simulink model "sevietta_devel_2017h"  (R2013a)
(part 6 of 31)

      | % if (strcmp(mode, 'one value') || strcmp(mode, 'fields of equal size')) && (length(current_widths) > 1),
      | %     error('Only one width may be specified for this mode.');
      | % elseif strcmp(mode, 'fields of arbitrary size')
      | %     current_names = textscan(strtrim(strrep(strrep(get_param(blk, 'names'), ']', ''), '[', '')), '%s');
      | %     current_names = current_names{1};
      | %     numios = length(current_names);
      | %     if length(current_widths) ~= numios,
      | %         error('%d field names specified, but %d widths?', numios, length(current_widths));
      | %     end
      | % end
      | % total_width = 0;
      | % for ctr = 1 : length(current_widths),
      | %     total_width = total_width + current_widths(ctr);
      | % end
      | % if total_width > 32,
      | %     error('Total width must be 32 or less, set to %d.', total_width);
      | % end
      mask Callback arith_types:
      | [numios, ~, ~, ~, current_types] = swreg_maskcheck(gcb);
      | % blk = gcb;
      | % mode = get_param(blk, 'mode');
      | % current_types = eval(get_param(blk, 'arith_types'));
      | % numios = length(current_types);
      | % if (strcmp(mode, 'one value') || strcmp(mode, 'fields of equal size')) && (length(current_types) > 1),
      | %     error('Only one type may be specified for this mode.');
      | % elseif strcmp(mode, 'fields of arbitrary size')
      | %     current_names = textscan(strtrim(strrep(strrep(get_param(blk, 'names'), ']', ''), '[', '')), '%s');
      | %     current_names = current_names{1};
      | %     numios = length(current_names);
      | %     if length(current_types) ~= numios,
      | %         error('%d field names specified, but %d types?', numios, length(current_types));
      | %     end
      | % end
      | problem = 0;
      | for ctr = 1 : numios,
      |     t = current_types(ctr);
      |     if (t < 0) || (t > 2),
      |         problem = t;
      |         ctr = numios + 1;
      |     end
      | end
      | if problem ~= 0,
      |     error('Type cannot be %i, must be 0, 1 or 2.', problem);
      | end
      mask Callback bin_pts:
      | swreg_maskcheck(gcb);
      | % blk = gcb;
      | % mode = get_param(blk, 'mode');
      | % current_bins = eval(get_param(blk, 'bin_pts'));
      | % if (strcmp(mode, 'one value') || strcmp(mode, 'fields of equal size')) && (length(current_bins) > 1),
      | %     error('Only one binary pt may be specified for this mode.');
      | % elseif strcmp(mode, 'fields of arbitrary size')
      | %     current_names = textscan(strtrim(strrep(strrep(get_param(blk, 'names'), ']', ''), '[', '')), '%s');
      | %     current_names = current_names{1};
      | %     numios = length(current_names);
      | %     if length(current_bins) ~= numios,
      | %         error('%d field names specified, but %d binary pts?', numios, length(current_bins));
      | %     end
      | % end
  packetizer : Subsystem
  packetizer1 : Subsystem
  packetizer2 : Subsystem
  packetizer3 : Subsystem
  pipeline1 : Subsystem  AncestorBlock=casper_library_delays/pipeline  mask(pipeline){latency=1}
      mask help:
      | An explicitly laid-out delay line to avoid mapping to SRL16s
      | for use in pipelining to help achieve timing closure.
      mask init:
      | pipeline_init(gcb,'latency',latency);
      settings: AttributesFormatString=Latency = %<latency>
      mask Display:
      | port_label('input', 1, 'd');
      | port_label('output', 1, 'q');
      | disp(['Z^-', num2str(latency)]);
  pipeline10 : Subsystem  AncestorBlock=casper_library_delays/pipeline  mask(pipeline){latency=1}
      mask help:
      | An explicitly laid-out delay line to avoid mapping to SRL16s
      | for use in pipelining to help achieve timing closure.
      mask init:
      | pipeline_init(gcb,'latency',latency);
      settings: AttributesFormatString=Latency = %<latency>
      mask Display:
      | port_label('input', 1, 'd');
      | port_label('output', 1, 'q');
      | disp(['Z^-', num2str(latency)]);
  pipeline11 : Subsystem  AncestorBlock=casper_library_delays/pipeline  mask(pipeline){latency=1}
      mask help:
      | An explicitly laid-out delay line to avoid mapping to SRL16s
      | for use in pipelining to help achieve timing closure.
      mask init:
      | pipeline_init(gcb,'latency',latency);
      settings: AttributesFormatString=Latency = %<latency>
      mask Display:
      | port_label('input', 1, 'd');
      | port_label('output', 1, 'q');
      | disp(['Z^-', num2str(latency)]);
  pipeline12 : Subsystem  AncestorBlock=casper_library_delays/pipeline  mask(pipeline){latency=1}
      mask help:
      | An explicitly laid-out delay line to avoid mapping to SRL16s
      | for use in pipelining to help achieve timing closure.
      mask init:
      | pipeline_init(gcb,'latency',latency);
      settings: AttributesFormatString=Latency = %<latency>
      mask Display:
      | port_label('input', 1, 'd');
      | port_label('output', 1, 'q');
      | disp(['Z^-', num2str(latency)]);
  pipeline13 : Subsystem  AncestorBlock=casper_library_delays/pipeline  mask(pipeline){latency=1}
      mask help:
      | An explicitly laid-out delay line to avoid mapping to SRL16s
      | for use in pipelining to help achieve timing closure.
      mask init:
      | pipeline_init(gcb,'latency',latency);
      settings: AttributesFormatString=Latency = %<latency>
      mask Display:
      | port_label('input', 1, 'd');
      | port_label('output', 1, 'q');
      | disp(['Z^-', num2str(latency)]);
  pipeline14 : Subsystem  AncestorBlock=casper_library_delays/pipeline  mask(pipeline){latency=1}
      mask help:
      | An explicitly laid-out delay line to avoid mapping to SRL16s
      | for use in pipelining to help achieve timing closure.
      mask init:
      | pipeline_init(gcb,'latency',latency);
      settings: AttributesFormatString=Latency = %<latency>
      mask Display:
      | port_label('input', 1, 'd');
      | port_label('output', 1, 'q');
      | disp(['Z^-', num2str(latency)]);
  pipeline15 : Subsystem  AncestorBlock=casper_library_delays/pipeline  mask(pipeline){latency=1}
      mask help:
      | An explicitly laid-out delay line to avoid mapping to SRL16s
      | for use in pipelining to help achieve timing closure.
      mask init:
      | pipeline_init(gcb,'latency',latency);
      settings: AttributesFormatString=Latency = %<latency>
      mask Display:
      | port_label('input', 1, 'd');
      | port_label('output', 1, 'q');
      | disp(['Z^-', num2str(latency)]);
  pipeline16 : Subsystem  AncestorBlock=casper_library_delays/pipeline  mask(pipeline){latency=1}
      mask help:
      | An explicitly laid-out delay line to avoid mapping to SRL16s
      | for use in pipelining to help achieve timing closure.
      mask init:
      | pipeline_init(gcb,'latency',latency);
      settings: AttributesFormatString=Latency = %<latency>
      mask Display:
      | port_label('input', 1, 'd');
      | port_label('output', 1, 'q');
      | disp(['Z^-', num2str(latency)]);
  pipeline17 : Subsystem  AncestorBlock=casper_library_delays/pipeline  mask(pipeline){latency=1}
      mask help:
      | An explicitly laid-out delay line to avoid mapping to SRL16s
      | for use in pipelining to help achieve timing closure.
      mask init:
      | pipeline_init(gcb,'latency',latency);
      settings: AttributesFormatString=Latency = %<latency>
      mask Display:
      | port_label('input', 1, 'd');
      | port_label('output', 1, 'q');
      | disp(['Z^-', num2str(latency)]);
  pipeline18 : Subsystem  AncestorBlock=casper_library_delays/pipeline  mask(pipeline){latency=1}
      mask help:
      | An explicitly laid-out delay line to avoid mapping to SRL16s
      | for use in pipelining to help achieve timing closure.
      mask init:
      | pipeline_init(gcb,'latency',latency);
      settings: AttributesFormatString=Latency = %<latency>
      mask Display:
      | port_label('input', 1, 'd');
      | port_label('output', 1, 'q');
      | disp(['Z^-', num2str(latency)]);
  pipeline19 : Subsystem  AncestorBlock=casper_library_delays/pipeline  mask(pipeline){latency=1}
      mask help:
      | An explicitly laid-out delay line to avoid mapping to SRL16s
      | for use in pipelining to help achieve timing closure.
      mask init:
      | pipeline_init(gcb,'latency',latency);
      settings: AttributesFormatString=Latency = %<latency>
      mask Display:
      | port_label('input', 1, 'd');
      | port_label('output', 1, 'q');
      | disp(['Z^-', num2str(latency)]);
  pipeline2 : Subsystem  AncestorBlock=casper_library_delays/pipeline  mask(pipeline){latency=1}
      mask help:
      | An explicitly laid-out delay line to avoid mapping to SRL16s
      | for use in pipelining to help achieve timing closure.
      mask init:
      | pipeline_init(gcb,'latency',latency);
      settings: AttributesFormatString=Latency = %<latency>
      mask Display:
      | port_label('input', 1, 'd');
      | port_label('output', 1, 'q');
      | disp(['Z^-', num2str(latency)]);
  pipeline20 : Subsystem  AncestorBlock=casper_library_delays/pipeline  mask(pipeline){latency=1}
      mask help:
      | An explicitly laid-out delay line to avoid mapping to SRL16s
      | for use in pipelining to help achieve timing closure.
      mask init:
      | pipeline_init(gcb,'latency',latency);
      settings: AttributesFormatString=Latency = %<latency>
      mask Display:
      | port_label('input', 1, 'd');
      | port_label('output', 1, 'q');
      | disp(['Z^-', num2str(latency)]);
  pipeline21 : Subsystem  AncestorBlock=casper_library_delays/pipeline  mask(pipeline){latency=1}
      mask help:
      | An explicitly laid-out delay line to avoid mapping to SRL16s
      | for use in pipelining to help achieve timing closure.
      mask init:
      | pipeline_init(gcb,'latency',latency);
      settings: AttributesFormatString=Latency = %<latency>
      mask Display:
      | port_label('input', 1, 'd');
      | port_label('output', 1, 'q');
      | disp(['Z^-', num2str(latency)]);
  pipeline22 : Subsystem  AncestorBlock=casper_library_delays/pipeline  mask(pipeline){latency=1}
      mask help:
      | An explicitly laid-out delay line to avoid mapping to SRL16s
      | for use in pipelining to help achieve timing closure.
      mask init:
      | pipeline_init(gcb,'latency',latency);
      settings: AttributesFormatString=Latency = %<latency>
      mask Display:
      | port_label('input', 1, 'd');
      | port_label('output', 1, 'q');
      | disp(['Z^-', num2str(latency)]);
  pipeline23 : Subsystem  AncestorBlock=casper_library_delays/pipeline  mask(pipeline){latency=1}
      mask help:
      | An explicitly laid-out delay line to avoid mapping to SRL16s
      | for use in pipelining to help achieve timing closure.
      mask init:
      | pipeline_init(gcb,'latency',latency);
      settings: AttributesFormatString=Latency = %<latency>
      mask Display:
      | port_label('input', 1, 'd');
      | port_label('output', 1, 'q');
      | disp(['Z^-', num2str(latency)]);
  pipeline24 : Subsystem  AncestorBlock=casper_library_delays/pipeline  mask(pipeline){latency=1}
      mask help:
      | An explicitly laid-out delay line to avoid mapping to SRL16s
      | for use in pipelining to help achieve timing closure.
      mask init:
      | pipeline_init(gcb,'latency',latency);
      settings: AttributesFormatString=Latency = %<latency>
      mask Display:
      | port_label('input', 1, 'd');
      | port_label('output', 1, 'q');
      | disp(['Z^-', num2str(latency)]);
  pipeline25 : Subsystem  AncestorBlock=casper_library_delays/pipeline  mask(pipeline){latency=1}
      mask help:
      | An explicitly laid-out delay line to avoid mapping to SRL16s
      | for use in pipelining to help achieve timing closure.
      mask init:
      | pipeline_init(gcb,'latency',latency);
      settings: AttributesFormatString=Latency = %<latency>
      mask Display:
      | port_label('input', 1, 'd');
      | port_label('output', 1, 'q');
      | disp(['Z^-', num2str(latency)]);
  pipeline26 : Subsystem  AncestorBlock=casper_library_delays/pipeline  mask(pipeline){latency=1}
      mask help:
      | An explicitly laid-out delay line to avoid mapping to SRL16s
      | for use in pipelining to help achieve timing closure.
      mask init:
      | pipeline_init(gcb,'latency',latency);
      settings: AttributesFormatString=Latency = %<latency>
      mask Display:
      | port_label('input', 1, 'd');
      | port_label('output', 1, 'q');
      | disp(['Z^-', num2str(latency)]);
  pipeline27 : Subsystem  AncestorBlock=casper_library_delays/pipeline  mask(pipeline){latency=1}
      mask help:
      | An explicitly laid-out delay line to avoid mapping to SRL16s
      | for use in pipelining to help achieve timing closure.
      mask init:
      | pipeline_init(gcb,'latency',latency);
      settings: AttributesFormatString=Latency = %<latency>
      mask Display:
      | port_label('input', 1, 'd');
      | port_label('output', 1, 'q');
      | disp(['Z^-', num2str(latency)]);
  pipeline28 : Subsystem  AncestorBlock=casper_library_delays/pipeline  mask(pipeline){latency=1}
      mask help:
      | An explicitly laid-out delay line to avoid mapping to SRL16s
      | for use in pipelining to help achieve timing closure.
      mask init:
      | pipeline_init(gcb,'latency',latency);
      settings: AttributesFormatString=Latency = %<latency>
      mask Display:
      | port_label('input', 1, 'd');
      | port_label('output', 1, 'q');
      | disp(['Z^-', num2str(latency)]);
  pipeline29 : Subsystem  AncestorBlock=casper_library_delays/pipeline  mask(pipeline){latency=1}
      mask help:
      | An explicitly laid-out delay line to avoid mapping to SRL16s
      | for use in pipelining to help achieve timing closure.
      mask init:
      | pipeline_init(gcb,'latency',latency);
      settings: AttributesFormatString=Latency = %<latency>
      mask Display:
      | port_label('input', 1, 'd');
      | port_label('output', 1, 'q');
      | disp(['Z^-', num2str(latency)]);
  pipeline3 : Subsystem  AncestorBlock=casper_library_delays/pipeline  mask(pipeline){latency=1}
      mask help:
      | An explicitly laid-out delay line to avoid mapping to SRL16s
      | for use in pipelining to help achieve timing closure.
      mask init:
      | pipeline_init(gcb,'latency',latency);
      settings: AttributesFormatString=Latency = %<latency>
      mask Display:
      | port_label('input', 1, 'd');
      | port_label('output', 1, 'q');
      | disp(['Z^-', num2str(latency)]);
  pipeline30 : Subsystem  AncestorBlock=casper_library_delays/pipeline  mask(pipeline){latency=1}
      mask help:
      | An explicitly laid-out delay line to avoid mapping to SRL16s
      | for use in pipelining to help achieve timing closure.
      mask init:
      | pipeline_init(gcb,'latency',latency);
      settings: AttributesFormatString=Latency = %<latency>
      mask Display:
      | port_label('input', 1, 'd');
      | port_label('output', 1, 'q');
      | disp(['Z^-', num2str(latency)]);
  pipeline31 : Subsystem  AncestorBlock=casper_library_delays/pipeline  mask(pipeline){latency=1}
      mask help:
      | An explicitly laid-out delay line to avoid mapping to SRL16s
      | for use in pipelining to help achieve timing closure.
      mask init:
      | pipeline_init(gcb,'latency',latency);
      settings: AttributesFormatString=Latency = %<latency>
      mask Display:
      | port_label('input', 1, 'd');
      | port_label('output', 1, 'q');
      | disp(['Z^-', num2str(latency)]);
  pipeline32 : Subsystem  AncestorBlock=casper_library_delays/pipeline  mask(pipeline){latency=1}
      mask help:
      | An explicitly laid-out delay line to avoid mapping to SRL16s
      | for use in pipelining to help achieve timing closure.
      mask init:
      | pipeline_init(gcb,'latency',latency);
      settings: AttributesFormatString=Latency = %<latency>
      mask Display:
      | port_label('input', 1, 'd');
      | port_label('output', 1, 'q');
      | disp(['Z^-', num2str(latency)]);
  pipeline33 : Subsystem  AncestorBlock=casper_library_delays/pipeline  mask(pipeline){latency=1}
      mask help:
      | An explicitly laid-out delay line to avoid mapping to SRL16s
      | for use in pipelining to help achieve timing closure.
      mask init:
      | pipeline_init(gcb,'latency',latency);
      settings: AttributesFormatString=Latency = %<latency>
      mask Display:
      | port_label('input', 1, 'd');
      | port_label('output', 1, 'q');
      | disp(['Z^-', num2str(latency)]);
  pipeline34 : Subsystem  AncestorBlock=casper_library_delays/pipeline  mask(pipeline){latency=1}
      mask help:
      | An explicitly laid-out delay line to avoid mapping to SRL16s
      | for use in pipelining to help achieve timing closure.
      mask init:
      | pipeline_init(gcb,'latency',latency);
      settings: AttributesFormatString=Latency = %<latency>
      mask Display:
      | port_label('input', 1, 'd');
      | port_label('output', 1, 'q');
      | disp(['Z^-', num2str(latency)]);
  pipeline35 : Subsystem  AncestorBlock=casper_library_delays/pipeline  mask(pipeline){latency=1}
      mask help:
      | An explicitly laid-out delay line to avoid mapping to SRL16s
      | for use in pipelining to help achieve timing closure.
      mask init:
      | pipeline_init(gcb,'latency',latency);
      settings: AttributesFormatString=Latency = %<latency>
      mask Display:
      | port_label('input', 1, 'd');
      | port_label('output', 1, 'q');
      | disp(['Z^-', num2str(latency)]);
  pipeline36 : Subsystem  AncestorBlock=casper_library_delays/pipeline  mask(pipeline){latency=1}
      mask help:
      | An explicitly laid-out delay line to avoid mapping to SRL16s
      | for use in pipelining to help achieve timing closure.
      mask init:
      | pipeline_init(gcb,'latency',latency);
      settings: AttributesFormatString=Latency = %<latency>
      mask Display:
      | port_label('input', 1, 'd');
      | port_label('output', 1, 'q');
      | disp(['Z^-', num2str(latency)]);
  pipeline37 : Subsystem  AncestorBlock=casper_library_delays/pipeline  mask(pipeline){latency=1}
      mask help:
      | An explicitly laid-out delay line to avoid mapping to SRL16s
      | for use in pipelining to help achieve timing closure.
      mask init:
      | pipeline_init(gcb,'latency',latency);
      settings: AttributesFormatString=Latency = %<latency>
      mask Display:
      | port_label('input', 1, 'd');
      | port_label('output', 1, 'q');
      | disp(['Z^-', num2str(latency)]);
  pipeline38 : Subsystem  AncestorBlock=casper_library_delays/pipeline  mask(pipeline){latency=1}
      mask help:
      | An explicitly laid-out delay line to avoid mapping to SRL16s
      | for use in pipelining to help achieve timing closure.
      mask init:
      | pipeline_init(gcb,'latency',latency);
      settings: AttributesFormatString=Latency = %<latency>
      mask Display:
      | port_label('input', 1, 'd');
      | port_label('output', 1, 'q');
      | disp(['Z^-', num2str(latency)]);
  pipeline39 : Subsystem  AncestorBlock=casper_library_delays/pipeline  mask(pipeline){latency=1}
      mask help:
      | An explicitly laid-out delay line to avoid mapping to SRL16s
      | for use in pipelining to help achieve timing closure.
      mask init:
      | pipeline_init(gcb,'latency',latency);
      settings: AttributesFormatString=Latency = %<latency>
      mask Display:
      | port_label('input', 1, 'd');
      | port_label('output', 1, 'q');
      | disp(['Z^-', num2str(latency)]);
  pipeline4 : Subsystem  AncestorBlock=casper_library_delays/pipeline  mask(pipeline){latency=1}
      mask help:
      | An explicitly laid-out delay line to avoid mapping to SRL16s
      | for use in pipelining to help achieve timing closure.
      mask init:
      | pipeline_init(gcb,'latency',latency);
      settings: AttributesFormatString=Latency = %<latency>
      mask Display:
      | port_label('input', 1, 'd');
      | port_label('output', 1, 'q');
      | disp(['Z^-', num2str(latency)]);
  pipeline40 : Subsystem  AncestorBlock=casper_library_delays/pipeline  mask(pipeline){latency=1}
      mask help:
      | An explicitly laid-out delay line to avoid mapping to SRL16s
      | for use in pipelining to help achieve timing closure.
      mask init:
      | pipeline_init(gcb,'latency',latency);
      settings: AttributesFormatString=Latency = %<latency>
      mask Display:
      | port_label('input', 1, 'd');
      | port_label('output', 1, 'q');
      | disp(['Z^-', num2str(latency)]);
  pipeline41 : Subsystem  AncestorBlock=casper_library_delays/pipeline  mask(pipeline){latency=1}
      mask help:
      | An explicitly laid-out delay line to avoid mapping to SRL16s
      | for use in pipelining to help achieve timing closure.
      mask init:
      | pipeline_init(gcb,'latency',latency);
      settings: AttributesFormatString=Latency = %<latency>
      mask Display:
      | port_label('input', 1, 'd');
      | port_label('output', 1, 'q');
      | disp(['Z^-', num2str(latency)]);
  pipeline42 : Subsystem  AncestorBlock=casper_library_delays/pipeline  mask(pipeline){latency=1}
      mask help:
      | An explicitly laid-out delay line to avoid mapping to SRL16s
      | for use in pipelining to help achieve timing closure.
      mask init:
      | pipeline_init(gcb,'latency',latency);
      settings: AttributesFormatString=Latency = %<latency>
      mask Display:
      | port_label('input', 1, 'd');
      | port_label('output', 1, 'q');
      | disp(['Z^-', num2str(latency)]);
  pipeline43 : Subsystem  AncestorBlock=casper_library_delays/pipeline  mask(pipeline){latency=1}
      mask help:
      | An explicitly laid-out delay line to avoid mapping to SRL16s
      | for use in pipelining to help achieve timing closure.
      mask init:
      | pipeline_init(gcb,'latency',latency);
      settings: AttributesFormatString=Latency = %<latency>
      mask Display:
      | port_label('input', 1, 'd');
      | port_label('output', 1, 'q');
      | disp(['Z^-', num2str(latency)]);
  pipeline44 : Subsystem  AncestorBlock=casper_library_delays/pipeline  mask(pipeline){latency=1}
      mask help:
      | An explicitly laid-out delay line to avoid mapping to SRL16s
      | for use in pipelining to help achieve timing closure.
      mask init:
      | pipeline_init(gcb,'latency',latency);
      settings: AttributesFormatString=Latency = %<latency>
      mask Display:
      | port_label('input', 1, 'd');
      | port_label('output', 1, 'q');
      | disp(['Z^-', num2str(latency)]);
  pipeline45 : Subsystem  AncestorBlock=casper_library_delays/pipeline  mask(pipeline){latency=1}
      mask help:
      | An explicitly laid-out delay line to avoid mapping to SRL16s
      | for use in pipelining to help achieve timing closure.
      mask init:
      | pipeline_init(gcb,'latency',latency);
      settings: AttributesFormatString=Latency = %<latency>
      mask Display:
      | port_label('input', 1, 'd');
      | port_label('output', 1, 'q');
      | disp(['Z^-', num2str(latency)]);
  pipeline46 : Subsystem  AncestorBlock=casper_library_delays/pipeline  mask(pipeline){latency=1}
      mask help:
      | An explicitly laid-out delay line to avoid mapping to SRL16s
      | for use in pipelining to help achieve timing closure.
      mask init:
      | pipeline_init(gcb,'latency',latency);
      settings: AttributesFormatString=Latency = %<latency>
      mask Display:
      | port_label('input', 1, 'd');
      | port_label('output', 1, 'q');
      | disp(['Z^-', num2str(latency)]);
  pipeline47 : Subsystem  AncestorBlock=casper_library_delays/pipeline  mask(pipeline){latency=1}
      mask help:
      | An explicitly laid-out delay line to avoid mapping to SRL16s
      | for use in pipelining to help achieve timing closure.
      mask init:
      | pipeline_init(gcb,'latency',latency);
      settings: AttributesFormatString=Latency = %<latency>
      mask Display:
      | port_label('input', 1, 'd');
      | port_label('output', 1, 'q');
      | disp(['Z^-', num2str(latency)]);
  pipeline48 : Subsystem  AncestorBlock=casper_library_delays/pipeline  mask(pipeline){latency=1}
      mask help:
      | An explicitly laid-out delay line to avoid mapping to SRL16s
      | for use in pipelining to help achieve timing closure.
      mask init:
      | pipeline_init(gcb,'latency',latency);
      settings: AttributesFormatString=Latency = %<latency>
      mask Display:
      | port_label('input', 1, 'd');
      | port_label('output', 1, 'q');
      | disp(['Z^-', num2str(latency)]);
  pipeline49 : Subsystem  AncestorBlock=casper_library_delays/pipeline  mask(pipeline){latency=1}
      mask help:
      | An explicitly laid-out delay line to avoid mapping to SRL16s
      | for use in pipelining to help achieve timing closure.
      mask init:
      | pipeline_init(gcb,'latency',latency);
      settings: AttributesFormatString=Latency = %<latency>
      mask Display:
      | port_label('input', 1, 'd');
      | port_label('output', 1, 'q');
      | disp(['Z^-', num2str(latency)]);
  pipeline5 : Subsystem  AncestorBlock=casper_library_delays/pipeline  mask(pipeline){latency=1}
      mask help:
      | An explicitly laid-out delay line to avoid mapping to SRL16s
      | for use in pipelining to help achieve timing closure.
      mask init:
      | pipeline_init(gcb,'latency',latency);
      settings: AttributesFormatString=Latency = %<latency>
      mask Display:
      | port_label('input', 1, 'd');
      | port_label('output', 1, 'q');
      | disp(['Z^-', num2str(latency)]);
  pipeline50 : Subsystem  AncestorBlock=casper_library_delays/pipeline  mask(pipeline){latency=1}
      mask help:
      | An explicitly laid-out delay line to avoid mapping to SRL16s
      | for use in pipelining to help achieve timing closure.
      mask init:
      | pipeline_init(gcb,'latency',latency);
      settings: AttributesFormatString=Latency = %<latency>
      mask Display:
      | port_label('input', 1, 'd');
      | port_label('output', 1, 'q');
      | disp(['Z^-', num2str(latency)]);
  pipeline51 : Subsystem  AncestorBlock=casper_library_delays/pipeline  mask(pipeline){latency=1}
      mask help:
      | An explicitly laid-out delay line to avoid mapping to SRL16s
      | for use in pipelining to help achieve timing closure.
      mask init:
      | pipeline_init(gcb,'latency',latency);
      settings: AttributesFormatString=Latency = %<latency>
      mask Display:
      | port_label('input', 1, 'd');
      | port_label('output', 1, 'q');
      | disp(['Z^-', num2str(latency)]);
  pipeline52 : Subsystem  AncestorBlock=casper_library_delays/pipeline  mask(pipeline){latency=1}
      mask help:
      | An explicitly laid-out delay line to avoid mapping to SRL16s
      | for use in pipelining to help achieve timing closure.
      mask init:
      | pipeline_init(gcb,'latency',latency);
      settings: AttributesFormatString=Latency = %<latency>
      mask Display:
      | port_label('input', 1, 'd');
      | port_label('output', 1, 'q');
      | disp(['Z^-', num2str(latency)]);
  pipeline53 : Subsystem  AncestorBlock=casper_library_delays/pipeline  mask(pipeline){latency=1}
      mask help:
      | An explicitly laid-out delay line to avoid mapping to SRL16s
      | for use in pipelining to help achieve timing closure.
      mask init:
      | pipeline_init(gcb,'latency',latency);
      settings: AttributesFormatString=Latency = %<latency>
      mask Display:
      | port_label('input', 1, 'd');
      | port_label('output', 1, 'q');
      | disp(['Z^-', num2str(latency)]);
  pipeline54 : Subsystem  AncestorBlock=casper_library_delays/pipeline  mask(pipeline){latency=1}
      mask help:
      | An explicitly laid-out delay line to avoid mapping to SRL16s
      | for use in pipelining to help achieve timing closure.
      mask init:
      | pipeline_init(gcb,'latency',latency);
      settings: AttributesFormatString=Latency = %<latency>
      mask Display:
      | port_label('input', 1, 'd');
      | port_label('output', 1, 'q');
      | disp(['Z^-', num2str(latency)]);
  pipeline55 : Subsystem  AncestorBlock=casper_library_delays/pipeline  mask(pipeline){latency=1}
      mask help:
      | An explicitly laid-out delay line to avoid mapping to SRL16s
      | for use in pipelining to help achieve timing closure.
      mask init:
      | pipeline_init(gcb,'latency',latency);
      settings: AttributesFormatString=Latency = %<latency>
      mask Display:
      | port_label('input', 1, 'd');
      | port_label('output', 1, 'q');
      | disp(['Z^-', num2str(latency)]);
  pipeline56 : Subsystem  AncestorBlock=casper_library_delays/pipeline  mask(pipeline){latency=1}
      mask help:
      | An explicitly laid-out delay line to avoid mapping to SRL16s
      | for use in pipelining to help achieve timing closure.
      mask init:
      | pipeline_init(gcb,'latency',latency);
      settings: AttributesFormatString=Latency = %<latency>
      mask Display:
      | port_label('input', 1, 'd');
      | port_label('output', 1, 'q');
      | disp(['Z^-', num2str(latency)]);
  pipeline57 : Subsystem  AncestorBlock=casper_library_delays/pipeline  mask(pipeline){latency=1}
      mask help:
      | An explicitly laid-out delay line to avoid mapping to SRL16s
      | for use in pipelining to help achieve timing closure.
      mask init:
      | pipeline_init(gcb,'latency',latency);
      settings: AttributesFormatString=Latency = %<latency>
      mask Display:
      | port_label('input', 1, 'd');
      | port_label('output', 1, 'q');
      | disp(['Z^-', num2str(latency)]);
  pipeline58 : Subsystem  AncestorBlock=casper_library_delays/pipeline  mask(pipeline){latency=1}
      mask help:
      | An explicitly laid-out delay line to avoid mapping to SRL16s
      | for use in pipelining to help achieve timing closure.
      mask init:
      | pipeline_init(gcb,'latency',latency);
      settings: AttributesFormatString=Latency = %<latency>
      mask Display:
      | port_label('input', 1, 'd');
      | port_label('output', 1, 'q');
      | disp(['Z^-', num2str(latency)]);
  pipeline59 : Subsystem  AncestorBlock=casper_library_delays/pipeline  mask(pipeline){latency=1}
      mask help:
      | An explicitly laid-out delay line to avoid mapping to SRL16s
      | for use in pipelining to help achieve timing closure.
      mask init:
      | pipeline_init(gcb,'latency',latency);
      settings: AttributesFormatString=Latency = %<latency>
      mask Display:
      | port_label('input', 1, 'd');
      | port_label('output', 1, 'q');
      | disp(['Z^-', num2str(latency)]);
  pipeline6 : Subsystem  AncestorBlock=casper_library_delays/pipeline  mask(pipeline){latency=1}
      mask help:
      | An explicitly laid-out delay line to avoid mapping to SRL16s
      | for use in pipelining to help achieve timing closure.
      mask init:
      | pipeline_init(gcb,'latency',latency);
      settings: AttributesFormatString=Latency = %<latency>
      mask Display:
      | port_label('input', 1, 'd');
      | port_label('output', 1, 'q');
      | disp(['Z^-', num2str(latency)]);
  pipeline60 : Subsystem  AncestorBlock=casper_library_delays/pipeline  mask(pipeline){latency=1}
      mask help:
      | An explicitly laid-out delay line to avoid mapping to SRL16s
      | for use in pipelining to help achieve timing closure.
      mask init:
      | pipeline_init(gcb,'latency',latency);
      settings: AttributesFormatString=Latency = %<latency>
      mask Display:
      | port_label('input', 1, 'd');
      | port_label('output', 1, 'q');
      | disp(['Z^-', num2str(latency)]);
  pipeline61 : Subsystem  AncestorBlock=casper_library_delays/pipeline  mask(pipeline){latency=1}
      mask help:
      | An explicitly laid-out delay line to avoid mapping to SRL16s
      | for use in pipelining to help achieve timing closure.
      mask init:
      | pipeline_init(gcb,'latency',latency);
      settings: AttributesFormatString=Latency = %<latency>
      mask Display:
      | port_label('input', 1, 'd');
      | port_label('output', 1, 'q');
      | disp(['Z^-', num2str(latency)]);
  pipeline62 : Subsystem  AncestorBlock=casper_library_delays/pipeline  mask(pipeline){latency=1}
      mask help:
      | An explicitly laid-out delay line to avoid mapping to SRL16s
      | for use in pipelining to help achieve timing closure.
      mask init:
      | pipeline_init(gcb,'latency',latency);
      settings: AttributesFormatString=Latency = %<latency>
      mask Display:
      | port_label('input', 1, 'd');
      | port_label('output', 1, 'q');
      | disp(['Z^-', num2str(latency)]);
  pipeline63 : Subsystem  AncestorBlock=casper_library_delays/pipeline  mask(pipeline){latency=1}
      mask help:
      | An explicitly laid-out delay line to avoid mapping to SRL16s
      | for use in pipelining to help achieve timing closure.
      mask init:
      | pipeline_init(gcb,'latency',latency);
      settings: AttributesFormatString=Latency = %<latency>
      mask Display:
      | port_label('input', 1, 'd');
      | port_label('output', 1, 'q');
      | disp(['Z^-', num2str(latency)]);
  pipeline64 : Subsystem  AncestorBlock=casper_library_delays/pipeline  mask(pipeline){latency=1}
      mask help:
      | An explicitly laid-out delay line to avoid mapping to SRL16s
      | for use in pipelining to help achieve timing closure.
      mask init:
      | pipeline_init(gcb,'latency',latency);
      settings: AttributesFormatString=Latency = %<latency>
      mask Display:
      | port_label('input', 1, 'd');
      | port_label('output', 1, 'q');
      | disp(['Z^-', num2str(latency)]);
  pipeline65 : Subsystem  AncestorBlock=casper_library_delays/pipeline  mask(pipeline){latency=1}
      mask help:
      | An explicitly laid-out delay line to avoid mapping to SRL16s
      | for use in pipelining to help achieve timing closure.
      mask init:
      | pipeline_init(gcb,'latency',latency);
      settings: AttributesFormatString=Latency = %<latency>
      mask Display:
      | port_label('input', 1, 'd');
      | port_label('output', 1, 'q');
      | disp(['Z^-', num2str(latency)]);
  pipeline66 : Subsystem  AncestorBlock=casper_library_delays/pipeline  mask(pipeline){latency=1}
      mask help:
      | An explicitly laid-out delay line to avoid mapping to SRL16s
      | for use in pipelining to help achieve timing closure.
      mask init:
      | pipeline_init(gcb,'latency',latency);
      settings: AttributesFormatString=Latency = %<latency>
      mask Display:
      | port_label('input', 1, 'd');
      | port_label('output', 1, 'q');
      | disp(['Z^-', num2str(latency)]);
  pipeline67 : Subsystem  AncestorBlock=casper_library_delays/pipeline  mask(pipeline){latency=1}
      mask help:
      | An explicitly laid-out delay line to avoid mapping to SRL16s
      | for use in pipelining to help achieve timing closure.
      mask init:
      | pipeline_init(gcb,'latency',latency);
      settings: AttributesFormatString=Latency = %<latency>
      mask Display:
      | port_label('input', 1, 'd');
      | port_label('output', 1, 'q');
      | disp(['Z^-', num2str(latency)]);
  pipeline68 : Subsystem  AncestorBlock=casper_library_delays/pipeline  mask(pipeline){latency=1}
      mask help:
      | An explicitly laid-out delay line to avoid mapping to SRL16s
      | for use in pipelining to help achieve timing closure.
      mask init:
      | pipeline_init(gcb,'latency',latency);
      settings: AttributesFormatString=Latency = %<latency>
      mask Display:
      | port_label('input', 1, 'd');
      | port_label('output', 1, 'q');
      | disp(['Z^-', num2str(latency)]);
  pipeline69 : Subsystem  AncestorBlock=casper_library_delays/pipeline  mask(pipeline){latency=1}
      mask help:
      | An explicitly laid-out delay line to avoid mapping to SRL16s
      | for use in pipelining to help achieve timing closure.
      mask init:
      | pipeline_init(gcb,'latency',latency);
      settings: AttributesFormatString=Latency = %<latency>
      mask Display:
      | port_label('input', 1, 'd');
      | port_label('output', 1, 'q');
      | disp(['Z^-', num2str(latency)]);
  pipeline7 : Subsystem  AncestorBlock=casper_library_delays/pipeline  mask(pipeline){latency=1}
      mask help:
      | An explicitly laid-out delay line to avoid mapping to SRL16s
      | for use in pipelining to help achieve timing closure.
      mask init:
      | pipeline_init(gcb,'latency',latency);
      settings: AttributesFormatString=Latency = %<latency>
      mask Display:
      | port_label('input', 1, 'd');
      | port_label('output', 1, 'q');
      | disp(['Z^-', num2str(latency)]);
  pipeline70 : Subsystem  AncestorBlock=casper_library_delays/pipeline  mask(pipeline){latency=1}
      mask help:
      | An explicitly laid-out delay line to avoid mapping to SRL16s
      | for use in pipelining to help achieve timing closure.
      mask init:
      | pipeline_init(gcb,'latency',latency);
      settings: AttributesFormatString=Latency = %<latency>
      mask Display:
      | port_label('input', 1, 'd');
      | port_label('output', 1, 'q');
      | disp(['Z^-', num2str(latency)]);
  pipeline71 : Subsystem  AncestorBlock=casper_library_delays/pipeline  mask(pipeline){latency=1}
      mask help:
      | An explicitly laid-out delay line to avoid mapping to SRL16s
      | for use in pipelining to help achieve timing closure.
      mask init:
      | pipeline_init(gcb,'latency',latency);
      settings: AttributesFormatString=Latency = %<latency>
      mask Display:
      | port_label('input', 1, 'd');
      | port_label('output', 1, 'q');
      | disp(['Z^-', num2str(latency)]);
  pipeline72 : Subsystem  AncestorBlock=casper_library_delays/pipeline  mask(pipeline){latency=1}
      mask help:
      | An explicitly laid-out delay line to avoid mapping to SRL16s
      | for use in pipelining to help achieve timing closure.
      mask init:
      | pipeline_init(gcb,'latency',latency);
      settings: AttributesFormatString=Latency = %<latency>
      mask Display:
      | port_label('input', 1, 'd');
      | port_label('output', 1, 'q');
      | disp(['Z^-', num2str(latency)]);
  pipeline73 : Subsystem  AncestorBlock=casper_library_delays/pipeline  mask(pipeline){latency=1}
      mask help:
      | An explicitly laid-out delay line to avoid mapping to SRL16s
      | for use in pipelining to help achieve timing closure.
      mask init:
      | pipeline_init(gcb,'latency',latency);
      settings: AttributesFormatString=Latency = %<latency>
      mask Display:
      | port_label('input', 1, 'd');
      | port_label('output', 1, 'q');
      | disp(['Z^-', num2str(latency)]);
  pipeline74 : Subsystem  AncestorBlock=casper_library_delays/pipeline  mask(pipeline){latency=1}
      mask help:
      | An explicitly laid-out delay line to avoid mapping to SRL16s
      | for use in pipelining to help achieve timing closure.
      mask init:
      | pipeline_init(gcb,'latency',latency);
      settings: AttributesFormatString=Latency = %<latency>
      mask Display:
      | port_label('input', 1, 'd');
      | port_label('output', 1, 'q');
      | disp(['Z^-', num2str(latency)]);
  pipeline75 : Subsystem  AncestorBlock=casper_library_delays/pipeline  mask(pipeline){latency=1}
      mask help:
      | An explicitly laid-out delay line to avoid mapping to SRL16s
      | for use in pipelining to help achieve timing closure.
      mask init:
      | pipeline_init(gcb,'latency',latency);
      settings: AttributesFormatString=Latency = %<latency>
      mask Display:
      | port_label('input', 1, 'd');
      | port_label('output', 1, 'q');
      | disp(['Z^-', num2str(latency)]);
  pipeline76 : Subsystem  AncestorBlock=casper_library_delays/pipeline  mask(pipeline){latency=1}
      mask help:
      | An explicitly laid-out delay line to avoid mapping to SRL16s
      | for use in pipelining to help achieve timing closure.
      mask init:
      | pipeline_init(gcb,'latency',latency);
      settings: AttributesFormatString=Latency = %<latency>
      mask Display:
      | port_label('input', 1, 'd');
      | port_label('output', 1, 'q');
      | disp(['Z^-', num2str(latency)]);
  pipeline77 : Subsystem  AncestorBlock=casper_library_delays/pipeline  mask(pipeline){latency=1}
      mask help:
      | An explicitly laid-out delay line to avoid mapping to SRL16s
      | for use in pipelining to help achieve timing closure.
      mask init:
      | pipeline_init(gcb,'latency',latency);
      settings: AttributesFormatString=Latency = %<latency>
      mask Display:
      | port_label('input', 1, 'd');
      | port_label('output', 1, 'q');
      | disp(['Z^-', num2str(latency)]);
  pipeline78 : Subsystem  AncestorBlock=casper_library_delays/pipeline  mask(pipeline){latency=1}
      mask help:
      | An explicitly laid-out delay line to avoid mapping to SRL16s
      | for use in pipelining to help achieve timing closure.
      mask init:
      | pipeline_init(gcb,'latency',latency);
      settings: AttributesFormatString=Latency = %<latency>
      mask Display:
      | port_label('input', 1, 'd');
      | port_label('output', 1, 'q');
      | disp(['Z^-', num2str(latency)]);
  pipeline79 : Subsystem  AncestorBlock=casper_library_delays/pipeline  mask(pipeline){latency=1}
      mask help:
      | An explicitly laid-out delay line to avoid mapping to SRL16s
      | for use in pipelining to help achieve timing closure.
      mask init:
      | pipeline_init(gcb,'latency',latency);
      settings: AttributesFormatString=Latency = %<latency>
      mask Display:
      | port_label('input', 1, 'd');
      | port_label('output', 1, 'q');
      | disp(['Z^-', num2str(latency)]);
  pipeline8 : Subsystem  AncestorBlock=casper_library_delays/pipeline  mask(pipeline){latency=1}
      mask help:
      | An explicitly laid-out delay line to avoid mapping to SRL16s
      | for use in pipelining to help achieve timing closure.
      mask init:
      | pipeline_init(gcb,'latency',latency);
      settings: AttributesFormatString=Latency = %<latency>
      mask Display:
      | port_label('input', 1, 'd');
      | port_label('output', 1, 'q');
      | disp(['Z^-', num2str(latency)]);
  pipeline80 : Subsystem  AncestorBlock=casper_library_delays/pipeline  mask(pipeline){latency=1}
      mask help:
      | An explicitly laid-out delay line to avoid mapping to SRL16s
      | for use in pipelining to help achieve timing closure.
      mask init:
      | pipeline_init(gcb,'latency',latency);
      settings: AttributesFormatString=Latency = %<latency>
      mask Display:
      | port_label('input', 1, 'd');
      | port_label('output', 1, 'q');
      | disp(['Z^-', num2str(latency)]);
  pipeline81 : Subsystem  AncestorBlock=casper_library_delays/pipeline  mask(pipeline){latency=1}
      mask help:
      | An explicitly laid-out delay line to avoid mapping to SRL16s
      | for use in pipelining to help achieve timing closure.
      mask init:
      | pipeline_init(gcb,'latency',latency);
      settings: AttributesFormatString=Latency = %<latency>
      mask Display:
      | port_label('input', 1, 'd');
      | port_label('output', 1, 'q');
      | disp(['Z^-', num2str(latency)]);
  pipeline82 : Subsystem  AncestorBlock=casper_library_delays/pipeline  mask(pipeline){latency=1}
      mask help:
      | An explicitly laid-out delay line to avoid mapping to SRL16s
      | for use in pipelining to help achieve timing closure.
      mask init:
      | pipeline_init(gcb,'latency',latency);
      settings: AttributesFormatString=Latency = %<latency>
      mask Display:
      | port_label('input', 1, 'd');
      | port_label('output', 1, 'q');
      | disp(['Z^-', num2str(latency)]);
  pipeline83 : Subsystem  AncestorBlock=casper_library_delays/pipeline  mask(pipeline){latency=1}
      mask help:
      | An explicitly laid-out delay line to avoid mapping to SRL16s
      | for use in pipelining to help achieve timing closure.
      mask init:
      | pipeline_init(gcb,'latency',latency);
      settings: AttributesFormatString=Latency = %<latency>
      mask Display:
      | port_label('input', 1, 'd');
      | port_label('output', 1, 'q');
      | disp(['Z^-', num2str(latency)]);
  pipeline84 : Subsystem  AncestorBlock=casper_library_delays/pipeline  mask(pipeline){latency=1}
      mask help:
      | An explicitly laid-out delay line to avoid mapping to SRL16s
      | for use in pipelining to help achieve timing closure.
      mask init:
      | pipeline_init(gcb,'latency',latency);
      settings: AttributesFormatString=Latency = %<latency>
      mask Display:
      | port_label('input', 1, 'd');
      | port_label('output', 1, 'q');
      | disp(['Z^-', num2str(latency)]);
  pipeline9 : Subsystem  AncestorBlock=casper_library_delays/pipeline  mask(pipeline){latency=1}
      mask help:
      | An explicitly laid-out delay line to avoid mapping to SRL16s
      | for use in pipelining to help achieve timing closure.
      mask init:
      | pipeline_init(gcb,'latency',latency);
      settings: AttributesFormatString=Latency = %<latency>
      mask Display:
      | port_label('input', 1, 'd');
      | port_label('output', 1, 'q');
      | disp(['Z^-', num2str(latency)]);
  regup1 : Subsystem
  regup10 : Subsystem
  regup11 : Subsystem
  regup12 : Subsystem
  regup13 : Subsystem
  regup14 : Subsystem
  regup15 : Subsystem
  regup16 : Subsystem
  regup17 : Subsystem
  regup2 : Subsystem
  regup3 : Subsystem
  regup4 : Subsystem
  regup5 : Subsystem
  regup6 : Subsystem
  regup7 : Subsystem
  regup8 : Subsystem
  regup9 : Subsystem
  roach_id : Subsystem  Tag=xps:sw_reg  AncestorBlock=xps_library/software_register  mask(swreg){mode=one value, io_dir=From Processor, io_delay=0, sample_period=1, names=reg, bitwidths=32, arith_types=0, bin_pts=0, sim_port=on, show_format=off}
      mask prompts: io_dir "I/O direction"; io_delay "I/O delay"; sample_period "Sample period"; names "Name:"; bitwidths "Bitwidth:"; arith_types "Type (ufix=0, fix=1, bool=2):"; bin_pts "Binary pt:"; sim_port "Provide sim input/output?"; show_format "Print format string?"
      mask init:
      | swreg_init(gcb)
      settings: AttributesFormatString=1input
      mask TypeOptions mode: one value | fields of equal size | fields of arbitrary size
      mask Callback mode: swreg_cb(gcb);
      mask TypeOptions io_dir: To Processor | From Processor
      mask Callback io_dir:
      | mask_enables = get_param(gcb, 'MaskEnables');
      | mask_names = get_param(gcb, 'MaskNames');
      | if strcmp(get_param(gcb, 'io_dir'), 'To Processor'),
      |     mask_enables{ismember(mask_names, 'sample_period')} = 'off';
      | else
      |     mask_enables{ismember(mask_names, 'sample_period')} = 'on';
      | end
      | set_param(gcb, 'MaskEnables', mask_enables);
      mask Callback bitwidths:
      | swreg_maskcheck(gcb);
      | % blk = gcb;
      | % mode = get_param(blk, 'mode');
      | % current_widths = eval(get_param(blk, 'bitwidths'));
      | % if (strcmp(mode, 'one value') || strcmp(mode, 'fields of equal size')) && (length(current_widths) > 1),
      | %     error('Only one width may be specified for this mode.');
      | % elseif strcmp(mode, 'fields of arbitrary size')
      | %     current_names = textscan(strtrim(strrep(strrep(get_param(blk, 'names'), ']', ''), '[', '')), '%s');
      | %     current_names = current_names{1};
      | %     numios = length(current_names);
      | %     if length(current_widths) ~= numios,
      | %         error('%d field names specified, but %d widths?', numios, length(current_widths));
      | %     end
      | % end
      | % total_width = 0;
      | % for ctr = 1 : length(current_widths),
      | %     total_width = total_width + current_widths(ctr);
      | % end
      | % if total_width > 32,
      | %     error('Total width must be 32 or less, set to %d.', total_width);
      | % end
      mask Callback arith_types:
      | [numios, ~, ~, ~, current_types] = swreg_maskcheck(gcb);
      | % blk = gcb;
      | % mode = get_param(blk, 'mode');
      | % current_types = eval(get_param(blk, 'arith_types'));
      | % numios = length(current_types);
      | % if (strcmp(mode, 'one value') || strcmp(mode, 'fields of equal size')) && (length(current_types) > 1),
      | %     error('Only one type may be specified for this mode.');
      | % elseif strcmp(mode, 'fields of arbitrary size')
      | %     current_names = textscan(strtrim(strrep(strrep(get_param(blk, 'names'), ']', ''), '[', '')), '%s');
      | %     current_names = current_names{1};
      | %     numios = length(current_names);
      | %     if length(current_types) ~= numios,
      | %         error('%d field names specified, but %d types?', numios, length(current_types));
      | %     end
      | % end
      | problem = 0;
      | for ctr = 1 : numios,
      |     t = current_types(ctr);
      |     if (t < 0) || (t > 2),
      |         problem = t;
      |         ctr = numios + 1;
      |     end
      | end
      | if problem ~= 0,
      |     error('Type cannot be %i, must be 0, 1 or 2.', problem);
      | end
      mask Callback bin_pts:
      | swreg_maskcheck(gcb);
      | % blk = gcb;
      | % mode = get_param(blk, 'mode');
      | % current_bins = eval(get_param(blk, 'bin_pts'));
      | % if (strcmp(mode, 'one value') || strcmp(mode, 'fields of equal size')) && (length(current_bins) > 1),
      | %     error('Only one binary pt may be specified for this mode.');
      | % elseif strcmp(mode, 'fields of arbitrary size')
      | %     current_names = textscan(strtrim(strrep(strrep(get_param(blk, 'names'), ']', ''), '[', '')), '%s');
      | %     current_names = current_names{1};
      | %     numios = length(current_names);
      | %     if length(current_bins) ~= numios,
      | %         error('%d field names specified, but %d binary pts?', numios, length(current_bins));
      | %     end
      | % end
  rx_ack{,1,4,6} (4 alike) : xbsIndex_r4/Constant  const=1  gui_display_data_type=Boolean  arith_type=Boolean  n_bits=32  bin_pt=0  preci_type=Single  exp_width=8  frac_width=24  explicit_period=on  period=1  equ=P=C  opselect=C  inp2=PCIN>>17  opr=+  inp1=P  carry=CIN  dbl_ovrd=off  block_type=constant
  rx_ack2 : xbsIndex_r4/Constant  const=0  gui_display_data_type=Fixed-point  arith_type=Unsigned  n_bits=16  bin_pt=0  preci_type=Single  exp_width=8  frac_width=24  explicit_period=on  period=1  equ=P=C  opselect=C  inp2=PCIN>>17  opr=+  inp1=P  carry=CIN  dbl_ovrd=off  block_type=constant
  rx_ack3 : xbsIndex_r4/Constant  const=1  gui_display_data_type=Fixed-point  arith_type=Unsigned  n_bits=16  bin_pt=0  preci_type=Single  exp_width=8  frac_width=24  explicit_period=on  period=1  equ=P=C  opselect=C  inp2=PCIN>>17  opr=+  inp1=P  carry=CIN  dbl_ovrd=off  block_type=constant
  rx_ack5 : xbsIndex_r4/Constant  const=1  gui_display_data_type=Fixed-point  arith_type=Unsigned  n_bits=16  bin_pt=0  preci_type=Single  exp_width=8  frac_width=24  explicit_period=on  period=1  equ=P=C  opselect=C  inp2=PCIN>>17  opr=+  inp1=P  carry=CIN  dbl_ovrd=off  block_type=constant
  rx_ack7 : xbsIndex_r4/Constant  const=1  gui_display_data_type=Fixed-point  arith_type=Unsigned  n_bits=16  bin_pt=0  preci_type=Single  exp_width=8  frac_width=24  explicit_period=on  period=1  equ=P=C  opselect=C  inp2=PCIN>>17  opr=+  inp1=P  carry=CIN  dbl_ovrd=off  block_type=constant
  tx_enable : Subsystem  Tag=xps:sw_reg  AncestorBlock=xps_library/software_register  mask(swreg){mode=one value, io_dir=From Processor, io_delay=0, sample_period=1, names=reg, bitwidths=8, arith_types=0, bin_pts=0, sim_port=on, show_format=off}
      mask prompts: io_dir "I/O direction"; io_delay "I/O delay"; sample_period "Sample period"; names "Name:"; bitwidths "Bitwidth:"; arith_types "Type (ufix=0, fix=1, bool=2):"; bin_pts "Binary pt:"; sim_port "Provide sim input/output?"; show_format "Print format string?"
      mask init:
      | swreg_init(gcb)
      settings: AttributesFormatString=1input
      mask TypeOptions mode: one value | fields of equal size | fields of arbitrary size
      mask Callback mode: swreg_cb(gcb);
      mask TypeOptions io_dir: To Processor | From Processor
      mask Callback io_dir:
      | mask_enables = get_param(gcb, 'MaskEnables');
      | mask_names = get_param(gcb, 'MaskNames');
      | if strcmp(get_param(gcb, 'io_dir'), 'To Processor'),
      |     mask_enables{ismember(mask_names, 'sample_period')} = 'off';
      | else
      |     mask_enables{ismember(mask_names, 'sample_period')} = 'on';
      | end
      | set_param(gcb, 'MaskEnables', mask_enables);
      mask Callback bitwidths:
      | swreg_maskcheck(gcb);
      | % blk = gcb;
      | % mode = get_param(blk, 'mode');
      | % current_widths = eval(get_param(blk, 'bitwidths'));
      | % if (strcmp(mode, 'one value') || strcmp(mode, 'fields of equal size')) && (length(current_widths) > 1),
      | %     error('Only one width may be specified for this mode.');
      | % elseif strcmp(mode, 'fields of arbitrary size')
      | %     current_names = textscan(strtrim(strrep(strrep(get_param(blk, 'names'), ']', ''), '[', '')), '%s');
      | %     current_names = current_names{1};
      | %     numios = length(current_names);
      | %     if length(current_widths) ~= numios,
      | %         error('%d field names specified, but %d widths?', numios, length(current_widths));
      | %     end
      | % end
      | % total_width = 0;
      | % for ctr = 1 : length(current_widths),
      | %     total_width = total_width + current_widths(ctr);
      | % end
      | % if total_width > 32,
      | %     error('Total width must be 32 or less, set to %d.', total_width);
      | % end
      mask Callback arith_types:
      | [numios, ~, ~, ~, current_types] = swreg_maskcheck(gcb);
      | % blk = gcb;
      | % mode = get_param(blk, 'mode');
      | % current_types = eval(get_param(blk, 'arith_types'));
      | % numios = length(current_types);
      | % if (strcmp(mode, 'one value') || strcmp(mode, 'fields of equal size')) && (length(current_types) > 1),
      | %     error('Only one type may be specified for this mode.');
      | % elseif strcmp(mode, 'fields of arbitrary size')
      | %     current_names = textscan(strtrim(strrep(strrep(get_param(blk, 'names'), ']', ''), '[', '')), '%s');
      | %     current_names = current_names{1};
      | %     numios = length(current_names);
      | %     if length(current_types) ~= numios,
      | %         error('%d field names specified, but %d types?', numios, length(current_types));
      | %     end
      | % end
      | problem = 0;
      | for ctr = 1 : numios,
      |     t = current_types(ctr);
      |     if (t < 0) || (t > 2),
      |         problem = t;
      |         ctr = numios + 1;
      |     end
      | end
      | if problem ~= 0,
      |     error('Type cannot be %i, must be 0, 1 or 2.', problem);
      | end
      mask Callback bin_pts:
      | swreg_maskcheck(gcb);
      | % blk = gcb;
      | % mode = get_param(blk, 'mode');
      | % current_bins = eval(get_param(blk, 'bin_pts'));
      | % if (strcmp(mode, 'one value') || strcmp(mode, 'fields of equal size')) && (length(current_bins) > 1),
      | %     error('Only one binary pt may be specified for this mode.');
      | % elseif strcmp(mode, 'fields of arbitrary size')
      | %     current_names = textscan(strtrim(strrep(strrep(get_param(blk, 'names'), ']', ''), '[', '')), '%s');
      | %     current_names = current_names{1};
      | %     numios = length(current_names);
      | %     if length(current_bins) ~= numios,
      | %         error('%d field names specified, but %d binary pts?', numios, length(current_bins));
      | %     end
      | % end
  tx_of_count{,1..7} (8 alike) : xbsIndex_r4/Counter  cnt_type=Free Running  cnt_to=21  operation=Up  start_count=0  cnt_by_val=1  arith_type=Unsigned  n_bits=18  bin_pt=0  load_pin=off  rst=on  en=on  explicit_period=on  period=1  dbl_ovrd=off  use_behavioral_HDL=off  implementation=Fabric  block_type=counter
      settings: block_version=11.4
  tx_rst : Subsystem  Tag=xps:sw_reg  AncestorBlock=xps_library/software_register  mask(swreg){mode=one value, io_dir=From Processor, io_delay=0, sample_period=1, names=reg, bitwidths=8, arith_types=0, bin_pts=0, sim_port=on, show_format=off}
      mask prompts: io_dir "I/O direction"; io_delay "I/O delay"; sample_period "Sample period"; names "Name:"; bitwidths "Bitwidth:"; arith_types "Type (ufix=0, fix=1, bool=2):"; bin_pts "Binary pt:"; sim_port "Provide sim input/output?"; show_format "Print format string?"
      mask init:
      | swreg_init(gcb)
      settings: AttributesFormatString=1input
      mask TypeOptions mode: one value | fields of equal size | fields of arbitrary size
      mask Callback mode: swreg_cb(gcb);
      mask TypeOptions io_dir: To Processor | From Processor
      mask Callback io_dir:
      | mask_enables = get_param(gcb, 'MaskEnables');
      | mask_names = get_param(gcb, 'MaskNames');
      | if strcmp(get_param(gcb, 'io_dir'), 'To Processor'),
      |     mask_enables{ismember(mask_names, 'sample_period')} = 'off';
      | else
      |     mask_enables{ismember(mask_names, 'sample_period')} = 'on';
      | end
      | set_param(gcb, 'MaskEnables', mask_enables);
      mask Callback bitwidths:
      | swreg_maskcheck(gcb);
      | % blk = gcb;
      | % mode = get_param(blk, 'mode');
      | % current_widths = eval(get_param(blk, 'bitwidths'));
      | % if (strcmp(mode, 'one value') || strcmp(mode, 'fields of equal size')) && (length(current_widths) > 1),
      | %     error('Only one width may be specified for this mode.');
      | % elseif strcmp(mode, 'fields of arbitrary size')
      | %     current_names = textscan(strtrim(strrep(strrep(get_param(blk, 'names'), ']', ''), '[', '')), '%s');
      | %     current_names = current_names{1};
      | %     numios = length(current_names);
      | %     if length(current_widths) ~= numios,
      | %         error('%d field names specified, but %d widths?', numios, length(current_widths));
      | %     end
      | % end
      | % total_width = 0;
      | % for ctr = 1 : length(current_widths),
      | %     total_width = total_width + current_widths(ctr);
      | % end
      | % if total_width > 32,
      | %     error('Total width must be 32 or less, set to %d.', total_width);
      | % end
      mask Callback arith_types:
      | [numios, ~, ~, ~, current_types] = swreg_maskcheck(gcb);
      | % blk = gcb;
      | % mode = get_param(blk, 'mode');
      | % current_types = eval(get_param(blk, 'arith_types'));
      | % numios = length(current_types);
      | % if (strcmp(mode, 'one value') || strcmp(mode, 'fields of equal size')) && (length(current_types) > 1),
      | %     error('Only one type may be specified for this mode.');
      | % elseif strcmp(mode, 'fields of arbitrary size')
      | %     current_names = textscan(strtrim(strrep(strrep(get_param(blk, 'names'), ']', ''), '[', '')), '%s');
      | %     current_names = current_names{1};
      | %     numios = length(current_names);
      | %     if length(current_types) ~= numios,
      | %         error('%d field names specified, but %d types?', numios, length(current_types));
      | %     end
      | % end
      | problem = 0;
      | for ctr = 1 : numios,
      |     t = current_types(ctr);
      |     if (t < 0) || (t > 2),
      |         problem = t;
      |         ctr = numios + 1;
      |     end
      | end
      | if problem ~= 0,
      |     error('Type cannot be %i, must be 0, 1 or 2.', problem);
      | end
      mask Callback bin_pts:
      | swreg_maskcheck(gcb);
      | % blk = gcb;
      | % mode = get_param(blk, 'mode');
      | % current_bins = eval(get_param(blk, 'bin_pts'));
      | % if (strcmp(mode, 'one value') || strcmp(mode, 'fields of equal size')) && (length(current_bins) > 1),
      | %     error('Only one binary pt may be specified for this mode.');
      | % elseif strcmp(mode, 'fields of arbitrary size')
      | %     current_names = textscan(strtrim(strrep(strrep(get_param(blk, 'names'), ']', ''), '[', '')), '%s');
      | %     current_names = current_names{1};
      | %     numios = length(current_names);
      | %     if length(current_bins) ~= numios,
      | %         error('%d field names specified, but %d binary pts?', numios, length(current_bins));
      | %     end
      | % end
  ws{0..1,12,16} (4 alike) : simulink/Sources/Repeating Sequence  rep_seq_t=v_time  rep_seq_y=v_chan_per_sub
  ws{5,8,10,13} (4 alike) : simulink/Sources/Repeating Sequence  rep_seq_t=v_time  rep_seq_y=v_stop_chan
  ws{2..3,11,15} (4 alike) : simulink/Sources/Repeating Sequence  rep_seq_t=v_time  rep_seq_y=v_subband
  ws{4,6..7,14} (4 alike) : simulink/Sources/Repeating Sequence  rep_seq_t=v_time  rep_seq_y=v_start_chan
  ws9 : simulink/Sources/Repeating Sequence  rep_seq_t=v_time  rep_seq_y=v_tx_en
  tag scope: chan_counter=global, gb00_eof=global, gb00_of=global, gb01_eof=global, gb01_of=global, gb02_eof=global, gb02_of=global, gb03_eof=global, gb03_of=global, gbe00_en=global, gbe00_rst=global, gbe01_en=global, gbe01_rst=global, gbe02_en=global, gbe02_rst=global, gbe03_en=global, gbe03_rst=global, led_tx1=global, led_tx2=global, led_tx3=global, led_tx=global, rst_seq_no=global, tx_port1=global, tx_port2=global, tx_port3=global, tx_port=global
  wires:
  In1/1 -> Terminator58/1
  [stop_chan] -> chan_start_stop0/3(stop_chan)
  [start_chan] -> chan_start_stop0/2(start_chan)
  gbe0_ip_port_bram/1(data_out) -> pipeline4/1(d)
  pipeline4/1(q) -> [tx_port]
  gbe0/3 -> [led_tx]
  gbe0/5 -> [gb00_of]
  gbe0_n_chan_per_sub/1(in_reg) -> Slice6/1
  gbe0_n_subband/1(in_reg) -> Slice5/1
  err_clear_sim4/1 -> roach_id/1(sim_1)
  roach_id/1(in_reg) -> Slice1/1
  pipeline7/1(q) -> [n_roach]
  gbe0_start_chan/1(in_reg) -> pipeline42/1(d)
  packetizer/2(tx_valid) -> Gateway Out7/1, Logical1/2
  packetizer/3(tx_eof) -> Gateway Out8/1, Logical2/2
  packetizer/1(tx_data) -> Gateway Out9/1, pipeline10/1(d)
  ip_we/1 -> gbe0_ip_addr_bram/3(we)
  packetizer/4(ip_addr_sel) -> Gateway Out10/1, [ip_addr_sel]
  ip_we1/1 -> gbe0_ip_addr_bram/2(data_in)
  gbe0_ip_addr_bram/1(data_out) -> [tx_dest_ip]
  [tx_dest_ip] -> pipeline12/1(d)
  [tx_port] -> pipeline13/1(d)
  rx_ack/1 -> pipeline16/1(d), pipeline15/1(d)
  [gbe00_en] -> Logical1/1
  Logical1/1 -> pipeline11/1(d)
  pipeline1/1(q) -> gbe0/1
  pipeline12/1(q) -> Gateway Out11/1, gbe0/4
  pipeline13/1(q) -> gbe0/5
  pipeline15/1(q) -> gbe0/7
  pipeline16/1(q) -> gbe0/8
  gbe0_linkup/1(sim_out) -> Terminator1/1
  pipeline17/1(q) -> gbe0_linkup/1(out_reg)
  gbe0/1 -> pipeline17/1(d)
  [gbe00_en] -> Logical2/1
  Logical2/1 -> [gb00_eof], pipeline14/1(d)
  Gateway Out4/1 -> Scope2/1  "data"
  Gateway Out2/1 -> Scope2/2  "valid"
  Gateway Out3/1 -> Scope2/3  "eof"
  gbe1/3 -> [led_tx1]
  gbe1/5 -> [gb01_of]
  packetizer1/2(tx_valid) -> Logical3/2, Gateway Out2/1
  packetizer1/3(tx_eof) -> Logical4/2, Gateway Out3/1
  packetizer1/1(tx_data) -> pipeline23/1(d), Gateway Out4/1
  [tx_dest_ip1] -> pipeline25/1(d)
  [tx_port1] -> pipeline26/1(d)
  rx_ack1/1 -> pipeline28/1(d), pipeline29/1(d)
  [gbe01_en] -> Logical3/1
  Logical3/1 -> pipeline24/1(d)
  pipeline22/1(q) -> gbe1/1
  pipeline25/1(q) -> gbe1/4
  pipeline26/1(q) -> gbe1/5
  pipeline28/1(q) -> gbe1/7
  pipeline29/1(q) -> gbe1/8
  gbe1_linkup/1(sim_out) -> Terminator5/1
  pipeline30/1(q) -> gbe1_linkup/1(out_reg)
  gbe1/1 -> pipeline30/1(d)
  [gbe01_en] -> Logical4/1
  Logical4/1 -> pipeline27/1(d), [gb01_eof]
  ip_we2/1 -> gbe1_ip_addr_bram/3(we)
  ip_we3/1 -> gbe1_ip_addr_bram/2(data_in)
  gbe1_ip_addr_bram/1(data_out) -> [tx_dest_ip1]
  gbe1_ip_port_bram/1(data_out) -> pipeline38/1(d)
  pipeline38/1(q) -> [tx_port1]
  gbe1_start_chan/1(in_reg) -> pipeline40/1(d)
  pipeline39/1(q) -> regup9/2(d_in)
  chan_start_stop1/1(valid) -> [chan_stst1]
  [new_fft] -> chan_start_stop1/1(rst)
  [start_chan1] -> chan_start_stop1/2(start_chan)
  [stop_chan1] -> chan_start_stop1/3(stop_chan)
  gbe1_n_subband/1(in_reg) -> Slice15/1
  ip_we4/1 -> gbe0_ip_port_bram/3(we)
  ip_we5/1 -> gbe0_ip_port_bram/2(data_in)
  ip_we6/1 -> gbe1_ip_port_bram/3(we)
  ip_we7/1 -> gbe1_ip_port_bram/2(data_in)
  [n_roach] -> packetizer/1(roach_id)
  [rst_seq_no] -> packetizer/2(rst)
  [n_chanps] -> packetizer/4(n_chanps)
  [n_subband] -> packetizer/5(n_subband)
  [fft_data] -> packetizer/6(data_in)
  [chan_stst0] -> packetizer/7(data_valid)
  rx_ack2/1 -> packetizer/8(gbe_id)
  [n_roach_tot] -> packetizer/9(header_spare)
  [start_chan] -> packetizer/10(first_chan)
  [n_roach_tot] -> packetizer1/9(header_spare)
  rx_ack3/1 -> packetizer1/8(gbe_id)
  [start_chan1] -> packetizer1/10(first_chan)
  [chan_stst1] -> packetizer1/7(data_valid)
  [fft_data] -> packetizer1/6(data_in)
  [n_subband1] -> packetizer1/5(n_subband)
  [n_chanps1] -> packetizer1/4(n_chanps)
  [new_fft] -> packetizer1/3(new_fft_win)
  [n_roach] -> packetizer1/1(roach_id)
  [rst_seq_no] -> packetizer1/2(rst)
  gbe1_n_chan_per_sub/1(in_reg) -> Slice8/1
  regup7/1(d_out) -> [start_chan]
  fft_length1/1 -> fft_count1/2(count_to)
  Constant8/1 -> fft_count1/3(en)
  fft_count1/1(new_count) -> Delay1/1  "end of window"
  fft_count1/2(count_out) -> [chan_counter]
  [sync_rnd] -> fft_count1/1(rst)
  Gateway Out9/1 -> Scope3/1  "data"
  Gateway Out7/1 -> Scope3/2  "valid"
  Gateway Out8/1 -> Scope3/3  "eof"
  Gateway Out10/1 -> Scope3/4  "ip_addr"
  chan_start_stop0/1(valid) -> [chan_stst0]
  ws4/1 -> gbe0_start_chan/1(sim_1)
  [new_fft] -> packetizer/3(new_fft_win)
  Delay1/1 -> [new_fft]
  [new_fft] -> chan_start_stop0/1(rst)
  cram/1(Out) -> Delay4/1
  err_clear_sim1/1 -> n_roach/1(sim_1)
  n_roach/1(in_reg) -> Slice9/1
  pipeline43/1(q) -> [n_roach_tot]
  pipeline8/1(q) -> regup7/2(d_in)
  regup9/1(d_out) -> [start_chan1]
  tx_enable/1(in_reg) -> pipeline9/1(d)
  Slice4/1 -> Delay10/1
  Slice3/1 -> Delay11/1
  ws9/1 -> tx_enable/1(sim_1)
  pipeline9/1(q) -> Slice17/1
  [ip_addr_sel] -> gbe0_ip_addr_bram/1(addr)
  [ip_addr_sel1] -> gbe1_ip_addr_bram/1(addr)
  [ip_addr_sel] -> gbe0_ip_port_bram/1(addr)
  [ip_addr_sel1] -> gbe1_ip_port_bram/1(addr)
  Delay10/1 -> [gbe00_en]
  Delay11/1 -> [gbe01_en]
  edge_detect2/1(out) -> [gbe03_rst], [gbe02_rst], [gbe01_rst], [gbe00_rst]
  [gbe00_rst] -> pipeline1/1(d)
  [gbe01_rst] -> pipeline22/1(d)
  [rst_seq_no] -> pipeline45/1(d)
  tx_of_count/1 -> pipeline18/1(d)
  gbe0_oflow_cnt/1(sim_out) -> Terminator6/1
  pipeline18/1(q) -> gbe0_oflow_cnt/1(out_reg)
  [gb00_of] -> tx_of_count/2
  pipeline45/1(q) -> tx_of_count/1
  [rst_seq_no] -> pipeline20/1(d)
  tx_of_count1/1 -> pipeline21/1(d)
  gbe0_eof_cnt/1(sim_out) -> Terminator4/1
  pipeline21/1(q) -> gbe0_eof_cnt/1(out_reg)
  [gb00_eof] -> tx_of_count1/2
  pipeline20/1(q) -> tx_of_count1/1
  [rst_seq_no] -> pipeline36/1(d)
  tx_of_count2/1 -> pipeline37/1(d)
  gbe1_oflow_cnt/1(sim_out) -> Terminator10/1
  pipeline37/1(q) -> gbe1_oflow_cnt/1(out_reg)
  [gb01_of] -> tx_of_count2/2
  pipeline36/1(q) -> tx_of_count2/1
  [rst_seq_no] -> pipeline33/1(d)
  tx_of_count3/1 -> pipeline35/1(d)
  gbe1_eof_cnt/1(sim_out) -> Terminator9/1
  pipeline35/1(q) -> gbe1_eof_cnt/1(out_reg)
  [gb01_eof] -> tx_of_count3/2
  pipeline33/1(q) -> tx_of_count3/1
  tx_rst/1(in_reg) -> Slice14/1
  regup1/1(d_out) -> edge_detect2/1(in)
  err_clear_sim7/1 -> tx_rst/1(sim_1)
  gbe0_stop_chan/1(in_reg) -> pipeline32/1(d)
  regup8/1(d_out) -> [stop_chan]
  ws5/1 -> gbe0_stop_chan/1(sim_1)
  pipeline31/1(q) -> regup8/2(d_in)
  ws0/1 -> gbe0_n_chan_per_sub/1(sim_1)
  ws1/1 -> gbe1_n_chan_per_sub/1(sim_1)
  ws2/1 -> gbe0_n_subband/1(sim_1)
  ws3/1 -> gbe1_n_subband/1(sim_1)
  pipeline2/1(q) -> regup3/2(d_in)
  regup3/1(d_out) -> [n_chanps]
  pipeline34/1(q) -> regup4/2(d_in)
  regup4/1(d_out) -> [n_chanps1]
  pipeline41/1(q) -> regup6/2(d_in)
  pipeline5/1(q) -> regup5/2(d_in)
  regup5/1(d_out) -> [n_subband]
  regup6/1(d_out) -> [n_subband1]
  Slice17/1 -> change_on_trig/3(d_in)
  [sync_rnd] -> regup3/1(sync_in)
  [sync_rnd] -> regup4/1(sync_in)
  [sync_rnd] -> regup5/1(sync_in)
  [sync_rnd] -> regup6/1(sync_in)
  gbe1_stop_chan/1(in_reg) -> pipeline6/1(d)
  pipeline3/1(q) -> regup10/2(d_in)
  ws8/1 -> gbe1_stop_chan/1(sim_1)
  regup10/1(d_out) -> [stop_chan1]
  ws7/1 -> gbe1_start_chan/1(sim_1)
  [new_fft] -> regup7/1(sync_in)
  [new_fft] -> regup8/1(sync_in)
  [new_fft] -> regup9/1(sync_in)
  [new_fft] -> regup10/1(sync_in)
  Gateway Out14/1 -> Scope6/1  "data"
  Gateway Out12/1 -> Scope6/2  "valid"
  Gateway Out13/1 -> Scope6/3  "eof"
  Gateway Out11/1 -> Scope6/4  "ip_addr"
  [sync_rnd] -> [rst_seq_no]
  [new_fft] -> regup1/1(sync_in)
  Slice14/1 -> pipeline19/1(d)
  pipeline19/1(q) -> regup1/2(d_in)
  pipeline11/1(q) -> Gateway Out12/1, gbe0/3
  pipeline14/1(q) -> gbe0/6, Gateway Out13/1
  pipeline24/1(q) -> gbe1/3
  pipeline27/1(q) -> gbe1/6
  pipeline10/1(q) -> Gateway Out14/1, gbe0/2
  pipeline23/1(q) -> gbe1/2
  [eq_out1] -> Delay7/1
  [eq_out] -> Delay6/1
  [eq_out2] -> Delay8/1
  [eq_out3] -> Delay9/1
  packetizer1/4(ip_addr_sel) -> [ip_addr_sel1]
  [every_second] -> change_on_trig/2(pps_in)
  [new_fft] -> change_on_trig/1(fft_sow_in)
  Slice15/1 -> pipeline41/1(d)
  Slice5/1 -> pipeline5/1(d)
  Slice8/1 -> pipeline34/1(d)
  Slice6/1 -> pipeline2/1(d)
  Slice9/1 -> pipeline43/1(d)
  Slice1/1 -> pipeline7/1(d)
  Slice18/1 -> pipeline31/1(d)
  Slice10/1 -> pipeline3/1(d)
  Slice2/1 -> pipeline39/1(d)
  Slice7/1 -> pipeline8/1(d)
  pipeline6/1(q) -> Slice10/1
  pipeline32/1(q) -> Slice18/1
  pipeline42/1(q) -> Slice7/1
  pipeline40/1(q) -> Slice2/1
  Delay7/1 -> cram/3(In3)
  Delay6/1 -> cram/4(In4)
  Delay8/1 -> cram/2(In2)
  Delay9/1 -> cram/1(In1)
  Gateway Out6/1 -> Scope1/1  "data"
  Gateway Out1/1 -> Scope1/2  "valid"
  Gateway Out5/1 -> Scope1/3  "eof"
  gbe2/3 -> [led_tx2]
  gbe2/5 -> [gb02_of]
  packetizer2/2(tx_valid) -> Gateway Out1/1, Logical5/2
  packetizer2/3(tx_eof) -> Gateway Out5/1, Logical6/2
  packetizer2/1(tx_data) -> Gateway Out6/1, pipeline46/1(d)
  [tx_dest_ip2] -> pipeline48/1(d)
  [tx_port2] -> pipeline49/1(d)
  rx_ack4/1 -> pipeline52/1(d), pipeline51/1(d)
  [gbe02_en] -> Logical5/1
  Logical5/1 -> pipeline47/1(d)
  gbe2_linkup/1(sim_out) -> Terminator2/1
  pipeline53/1(q) -> gbe2_linkup/1(out_reg)
  gbe2/1 -> pipeline53/1(d)
  [gbe02_en] -> Logical6/1
  Logical6/1 -> [gb02_eof], pipeline50/1(d)
  [n_roach_tot] -> packetizer2/9(header_spare)
  rx_ack5/1 -> packetizer2/8(gbe_id)
  [start_chan2] -> packetizer2/10(first_chan)
  [chan_stst2] -> packetizer2/7(data_valid)
  [fft_data] -> packetizer2/6(data_in)
  [n_subband2] -> packetizer2/5(n_subband)
  [n_chanps2] -> packetizer2/4(n_chanps)
  [new_fft] -> packetizer2/3(new_fft_win)
  [n_roach] -> packetizer2/1(roach_id)
  [rst_seq_no] -> packetizer2/2(rst)
  [gbe02_rst] -> pipeline44/1(d)
  packetizer2/4(ip_addr_sel) -> [ip_addr_sel2]
  ip_we8/1 -> gbe2_ip_addr_bram/3(we)
  ip_we9/1 -> gbe2_ip_addr_bram/2(data_in)
  gbe2_ip_addr_bram/1(data_out) -> [tx_dest_ip2]
  gbe2_ip_port_bram/1(data_out) -> pipeline54/1(d)
  pipeline54/1(q) -> [tx_port2]
  ip_we10/1 -> gbe2_ip_port_bram/3(we)
  ip_we11/1 -> gbe2_ip_port_bram/2(data_in)
  [ip_addr_sel2] -> gbe2_ip_addr_bram/1(addr)
  [ip_addr_sel2] -> gbe2_ip_port_bram/1(addr)
  gbe2_start_chan/1(in_reg) -> pipeline57/1(d)
  pipeline56/1(q) -> regup11/2(d_in)
  regup11/1(d_out) -> [start_chan2]
  gbe2_stop_chan/1(in_reg) -> pipeline58/1(d)
  pipeline55/1(q) -> regup2/2(d_in)
  ws10/1 -> gbe2_stop_chan/1(sim_1)
  regup2/1(d_out) -> [stop_chan2]
  ws6/1 -> gbe2_start_chan/1(sim_1)
  [new_fft] -> regup11/1(sync_in)
  [new_fft] -> regup2/1(sync_in)
  Slice16/1 -> pipeline55/1(d)
  Slice11/1 -> pipeline56/1(d)
  pipeline58/1(q) -> Slice16/1
  pipeline57/1(q) -> Slice11/1
  gbe2_n_subband/1(in_reg) -> Slice12/1
  ws11/1 -> gbe2_n_subband/1(sim_1)
  pipeline59/1(q) -> regup12/2(d_in)
  regup12/1(d_out) -> [n_subband2]
  [sync_rnd] -> regup12/1(sync_in)
  Slice12/1 -> pipeline59/1(d)
  gbe2_n_chan_per_sub/1(in_reg) -> Slice13/1
  ws12/1 -> gbe2_n_chan_per_sub/1(sim_1)
  pipeline60/1(q) -> regup13/2(d_in)
  regup13/1(d_out) -> [n_chanps2]
  [sync_rnd] -> regup13/1(sync_in)
  Slice13/1 -> pipeline60/1(d)
  chan_start_stop2/1(valid) -> [chan_stst2]
  [new_fft] -> chan_start_stop2/1(rst)
  [start_chan2] -> chan_start_stop2/2(start_chan)
  [stop_chan2] -> chan_start_stop2/3(stop_chan)
  Slice19/1 -> Delay2/1
  Delay2/1 -> [gbe02_en]
  [rst_seq_no] -> pipeline63/1(d)
  tx_of_count4/1 -> pipeline64/1(d)
  gbe2_oflow_cnt/1(sim_out) -> Terminator3/1
  pipeline64/1(q) -> gbe2_oflow_cnt/1(out_reg)
  [gb02_of] -> tx_of_count4/2
  pipeline63/1(q) -> tx_of_count4/1
  [rst_seq_no] -> pipeline61/1(d)
  tx_of_count5/1 -> pipeline62/1(d)
  gbe2_eof_cnt/1(sim_out) -> Terminator7/1
  pipeline62/1(q) -> gbe2_eof_cnt/1(out_reg)
  [gb02_eof] -> tx_of_count5/2
  pipeline61/1(q) -> tx_of_count5/1
  pipeline46/1(q) -> gbe2/2
  pipeline47/1(q) -> gbe2/3
  pipeline48/1(q) -> gbe2/4
  pipeline49/1(q) -> gbe2/5
  pipeline44/1(q) -> gbe2/1
  pipeline50/1(q) -> gbe2/6
  pipeline51/1(q) -> gbe2/7
  pipeline52/1(q) -> gbe2/8
  Gateway Out17/1 -> Scope4/1  "data"
  Gateway Out15/1 -> Scope4/2  "valid"
  Gateway Out16/1 -> Scope4/3  "eof"
  gbe3/3 -> [led_tx3]
  gbe3/5 -> [gb03_of]
  packetizer3/2(tx_valid) -> Logical7/2, Gateway Out15/1
  packetizer3/3(tx_eof) -> Logical8/2, Gateway Out16/1
  packetizer3/1(tx_data) -> pipeline66/1(d), Gateway Out17/1
  [tx_dest_ip3] -> pipeline68/1(d)
  [tx_port3] -> pipeline69/1(d)
  rx_ack6/1 -> pipeline71/1(d), pipeline72/1(d)
  [gbe03_en] -> Logical7/1
  Logical7/1 -> pipeline67/1(d)
  gbe3_linkup/1(sim_out) -> Terminator8/1
  pipeline73/1(q) -> gbe3_linkup/1(out_reg)
  gbe3/1 -> pipeline73/1(d)
  [gbe03_en] -> Logical8/1
  Logical8/1 -> pipeline70/1(d), [gb03_eof]
  [n_roach_tot] -> packetizer3/9(header_spare)
  rx_ack7/1 -> packetizer3/8(gbe_id)
  [start_chan3] -> packetizer3/10(first_chan)
  [chan_stst3] -> packetizer3/7(data_valid)
  [fft_data] -> packetizer3/6(data_in)
  [n_subband3] -> packetizer3/5(n_subband)
  [n_chanps3] -> packetizer3/4(n_chanps)
  [new_fft] -> packetizer3/3(new_fft_win)
  [n_roach] -> packetizer3/1(roach_id)
  [rst_seq_no] -> packetizer3/2(rst)
  [gbe03_rst] -> pipeline65/1(d)
  packetizer3/4(ip_addr_sel) -> [ip_addr_sel3]
  pipeline66/1(q) -> gbe3/2
  pipeline67/1(q) -> gbe3/3
  pipeline68/1(q) -> gbe3/4
  pipeline69/1(q) -> gbe3/5
  pipeline65/1(q) -> gbe3/1
  pipeline70/1(q) -> gbe3/6
  pipeline71/1(q) -> gbe3/7
  pipeline72/1(q) -> gbe3/8
  chan_start_stop3/1(valid) -> [chan_stst3]
  [new_fft] -> chan_start_stop3/1(rst)
  [start_chan3] -> chan_start_stop3/2(start_chan)
  [stop_chan3] -> chan_start_stop3/3(stop_chan)
  gbe3_start_chan/1(in_reg) -> pipeline76/1(d)
  pipeline75/1(q) -> regup14/2(d_in)
  regup14/1(d_out) -> [start_chan3]
  gbe3_stop_chan/1(in_reg) -> pipeline77/1(d)
  pipeline74/1(q) -> regup15/2(d_in)
  ws13/1 -> gbe3_stop_chan/1(sim_1)
  regup15/1(d_out) -> [stop_chan3]
  ws14/1 -> gbe3_start_chan/1(sim_1)
  [new_fft] -> regup14/1(sync_in)
  [new_fft] -> regup15/1(sync_in)
  Slice21/1 -> pipeline74/1(d)
  Slice20/1 -> pipeline75/1(d)
  pipeline77/1(q) -> Slice21/1
  pipeline76/1(q) -> Slice20/1
  ip_we14/1 -> gbe3_ip_addr_bram/3(we)
  ip_we15/1 -> gbe3_ip_addr_bram/2(data_in)
  gbe3_ip_addr_bram/1(data_out) -> [tx_dest_ip3]
  gbe3_ip_port_bram/1(data_out) -> pipeline78/1(d)
  pipeline78/1(q) -> [tx_port3]
  ip_we12/1 -> gbe3_ip_port_bram/3(we)
  ip_we13/1 -> gbe3_ip_port_bram/2(data_in)
  [ip_addr_sel2] -> gbe3_ip_addr_bram/1(addr)
  [ip_addr_sel2] -> gbe3_ip_port_bram/1(addr)
  [rst_seq_no] -> pipeline81/1(d)
  tx_of_count6/1 -> pipeline82/1(d)
  gbe3_oflow_cnt/1(sim_out) -> Terminator11/1
  pipeline82/1(q) -> gbe3_oflow_cnt/1(out_reg)
  [gb03_of] -> tx_of_count6/2
  pipeline81/1(q) -> tx_of_count6/1
  [rst_seq_no] -> pipeline79/1(d)
  tx_of_count7/1 -> pipeline80/1(d)
  gbe3_eof_cnt/1(sim_out) -> Terminator12/1
  pipeline80/1(q) -> gbe3_eof_cnt/1(out_reg)
  [gb03_eof] -> tx_of_count7/2
  pipeline79/1(q) -> tx_of_count7/1
  gbe3_n_subband/1(in_reg) -> Slice22/1
  ws15/1 -> gbe3_n_subband/1(sim_1)
  pipeline83/1(q) -> regup16/2(d_in)
  regup16/1(d_out) -> [n_subband3]
  [sync_rnd] -> regup16/1(sync_in)
  Slice22/1 -> pipeline83/1(d)
  change_on_trig/1(d_out) -> Slice23/1, Slice19/1, Slice3/1, Slice4/1
  Slice23/1 -> Delay3/1
  Delay3/1 -> [gbe03_en]
  gbe3_n_chan_per_sub/1(in_reg) -> Slice24/1
  ws16/1 -> gbe3_n_chan_per_sub/1(sim_1)
  pipeline84/1(q) -> regup17/2(d_in)
  regup17/1(d_out) -> [n_chanps3]
  [sync_rnd] -> regup17/1(sync_in)
  Slice24/1 -> pipeline84/1(d)
  Delay4/1 -> [fft_data]
